simulink model "PhyMtrCtrl"  (R2023b)
settings: Solver=VariableStepAuto  StartTime=0.0  StopTime=10.0  RelTol=1e-3
values from neighbouring files (symbols this model uses):
  B = 0.001889    [MtrCtrl_v01.sldd]    (also in PICal.m; PMSM.m = Simulink.Parameter)
  C_LUT_AngleTable_sng_Null = saveVarsMat.C_LUT_AngleTable_sng_Null    [AngleTable.m]    (also in PMSM.m)
  C_LUT_SinTable_sng_Null = saveVarsMat.C_LUT_SinTable_sng_Null    [AngleTable.m]    (also in PMSM.m)
  C_MATH_OneOverSqrtThree_s32n31_Null = Simulink.Parameter    [PMSM.m]
  C_MATH_Pi_u32n30_Null = Simulink.Parameter    [PMSM.m]
  C_MATH_SqrtThreeOverThree_s32n31_Null = Simulink.Parameter    [PMSM.m]
  C_PMSM_CurQKi_u32n31_null = Simulink.Parameter    [PMSM.m]
  C_PMSM_CurQKp_u32n31_null = Simulink.Parameter    [PMSM.m]
  C_PMSM_Flux_u32n32_Vs = Simulink.Parameter    [PMSM.m]
  Flux = 0.192    [MtrCtrl_v01.sldd]    (also in PICal.m; PMSM.m)
  IBase_A = 2000.0    [MtrCtrl_v01.sldd]    (also in PICal.m = 300; PMSM.m = Simulink.Parameter)
  J = 0.011    [MtrCtrl_v01.sldd]    (also in PICal.m; PMSM.m)
  K_SVM_DefultDuty_s32n31_Null = Simulink.Parameter    [PMSM.m]
  KCCM_VirPosn_flg = 0.0    [MtrCtrl_v01.sldd]    (also in PMSM.m = Simulink.Parameter)
  KCCM_VoltModeEna_Flg = 0.0    [MtrCtrl_v01.sldd]    (also in PMSM.m = Simulink.Parameter)
  Kis = 114583.3333333333    [MtrCtrl_v01.sldd]    (also in PICal.m = 114583.333333; PMSM.m = 114583.333333)
  Kt = 1.1520000000000001    [MtrCtrl_v01.sldd]    (also in PICal.m = 1.152; PMSM.m = 1.152)
  Ld = 80e-6    (= 8e-05)    [FluxweakingGen.m]    (also in IEHB_MAPGenerationtest.m = 6.8e-05; MtrCtrl_v01.sldd = 0.000635; PICal.m = 0.000635; PMSM.m = Simulink.Parameter)
  LPF_coefg = 0.01    [MtrCtrl_v01.sldd]    (also in PMSM.m = Simulink.Parameter)
  Lq = 80e-6    (= 8e-05)    [FluxweakingGen.m]    (also in IEHB_MAPGenerationtest.m = 6e-05; MtrCtrl_v01.sldd = 0.000685; PICal.m = 0.000635; PMSM.m = Simulink.Parameter)
  Ls = 0.000635    [MtrCtrl_v01.sldd]    (also in PICal.m; PMSM.m)
  OneOverUBase_V = Simulink.Parameter    [PMSM.m]
  Pp = 4.0    [MtrCtrl_v01.sldd]    (also in PICal.m = 4; PMSM.m = Simulink.Parameter)
  Rs = 0.03    [FluxweakingGen.m]    (also in MtrCtrl_v01.sldd = 0.05; PICal.m = 0.05; PMSM.m = Simulink.Parameter)
  SecPerRnd = 0.6    [MtrCtrl_v01.sldd]    (also in PMSM.m = Simulink.Parameter)
  sinTable = 0.0015339801862847655 0.0015339807878856412 0.0030679567629659761 0.0030679615757712823 0.0046019261204485705 0.0046019423636569235 0.0061358846491544753 0.0061359231515425647 0.007669828739531097 0.0076699039394282058 0.00920375478205982 0.009203884727313847 0.010737659167264491 0.010737865515199488 0.012271538285719925 0.012271846303085129 0.013805388528060391 0.013805827090970771 0.015339206284    [MtrCtrl_v01.sldd]    (also in SinLut.m = zeros(2,TableSize))
  SMOGain_V = 323.31615074619043    [MtrCtrl_v01.sldd]    (also in PMSM.m = Simulink.Parameter)
  Ts = 0.0001    [MtrCtrl_v01.sldd]    (also in PICal.m; PMSM.m = Simulink.Parameter)
  UBase_V = 600.0    [MtrCtrl_v01.sldd]    (also in PICal.m = 600; PMSM.m = Simulink.Parameter)
  wmBase_rps = 314.15926535897933    [MtrCtrl_v01.sldd]    (also in PICal.m = 314.159265359; PMSM.m = Simulink.Parameter)
undefined symbols (not defined in the file or in its folder): C_PMSM_Ls_pu, C_PMSM_PolePairs_u8_Null, DiscIntNeverNeededParam
libraries: ee_lib x16, simulink x10, nesl_utility x6, spsVoltageMeasurementLib x6, spsCurrentMeasurementLib x3, spsSeriesRLCBranchLib x3, simulink_extras x2, fl_lib x2, sdl_lib x1, eePmsmFwController x1, slpidlib x1, spspowerguiLib x1
(part 2 of 3)

== system PhyMtrCtrl/CurLpCtrl/InversePark ==
  D : Inport  OutDataTypeStr=fixdt(1,32,31)
  Q : Inport  Port=2  OutDataTypeStr=fixdt(1,32,31)
  SinTheta : Inport  Port=3  OutDataTypeStr=fixdt(1,32,30)
  CosTheta : Inport  Port=4  OutDataTypeStr=fixdt(1,32,30)
  Scope : Scope  NumInputPorts=2
  dcos : Product  OutDataTypeStr=fixdt(1,32,31)  RndMeth=Simplest
  dsin : Product  OutDataTypeStr=fixdt(1,32,31)  RndMeth=Simplest
  qcos : Product  OutDataTypeStr=fixdt(1,32,31)  RndMeth=Simplest
  qsin : Product  OutDataTypeStr=fixdt(1,32,31)  RndMeth=Simplest
  sum_alpha : Sum  Inputs=|+-  OutDataTypeStr=fixdt(1,32,31)  RndMeth=Simplest
  sum_beta : Sum  Inputs=|++  OutDataTypeStr=fixdt(1,32,31)  RndMeth=Simplest
  Alpha : Outport
  Beta : Outport  Port=2
  wires:
  sum_alpha/1 -> Scope/1, Alpha/1
  sum_beta/1 -> Scope/2, Beta/1
  dsin/1 -> sum_beta/2
  qcos/1 -> sum_beta/1
  CosTheta/1 -> dcos/2, qcos/2
  qsin/1 -> sum_alpha/2
  SinTheta/1 -> qsin/2, dsin/2
  Q/1 -> qcos/1, qsin/1
  dcos/1 -> sum_alpha/1
  D/1 -> dsin/1, dcos/1

== system PhyMtrCtrl/CurLpCtrl/ParkTF ==
  I_alpha : Inport  OutDataTypeStr=fixdt(1,32,31)
  I_beta : Inport  Port=2  OutDataTypeStr=fixdt(1,32,31)
  SinTheta : Inport  Port=3  OutDataTypeStr=fixdt(1,32,30)
  CosTheta : Inport  Port=4  OutDataTypeStr=fixdt(1,32,30)
  Add : Sum  OutDataTypeStr=fixdt(1,32,31)
  Add1 : Sum  Inputs=+-  OutDataTypeStr=fixdt(1,32,31)
  Product{,1..3} (4 alike) : Product  OutDataTypeStr=fixdt(1,32,31)
  Scope : Scope  NumInputPorts=2
  CurD : Outport
  CurQ : Outport  Port=2
  wires:
  Product/1 -> Add/1
  Product1/1 -> Add/2
  Add/1 -> Scope/1, CurD/1
  Add1/1 -> Scope/2, CurQ/1
  Product3/1 -> Add1/1
  Product2/1 -> Add1/2
  I_alpha/1 -> Product2/1, Product/1
  SinTheta/1 -> Product2/2, Product1/2
  I_beta/1 -> Product1/1, Product3/1
  CosTheta/1 -> Product/2, Product3/2

== system PhyMtrCtrl/CurLpCtrl/PhaseCut ==
  In1 : Inport  OutDataTypeStr=fixdt(1,32,4)
  In2 : Inport  Port=2  OutDataTypeStr=fixdt(0,32,33)
  In3 : Inport  Port=3  OutDataTypeStr=fixdt(0,32,33)
  In4 : Inport  Port=4  OutDataTypeStr=fixdt(0,32,33)
  Constant5 : Constant  Value=0.5  OutDataTypeStr=fixdt(0,32,32)
  Constant6 : Constant  Value=0.0  OutDataTypeStr=fixdt(1,32,4)
  Constant7 : Constant  Value=0.00  OutDataTypeStr=fixdt(1,32,4)
  Switch2 : Switch  Criteria=u2 > Threshold  OutDataTypeStr=fixdt(0,32,33)  SaturateOnIntegerOverflow=off  InputSameDT=off
  Switch3 : Switch  Criteria=u2 > Threshold  OutDataTypeStr=fixdt(0,32,33)  SaturateOnIntegerOverflow=off  InputSameDT=off
  Switch4 : Switch  Criteria=u2 > Threshold  OutDataTypeStr=fixdt(0,32,33)  SaturateOnIntegerOverflow=off  InputSameDT=off
  Out1 : Outport
  Out2 : Outport  Port=2
  Out3 : Outport  Port=3
  wires:
  Switch4/1 -> Out3/1
  Constant7/1 -> Switch4/1
  In2/1 -> Switch2/3
  In1/1 -> Switch2/2, Switch3/2, Switch4/2
  Constant5/1 -> Switch2/1
  Switch2/1 -> Out1/1
  Constant6/1 -> Switch3/1
  Switch3/1 -> Out2/1
  In4/1 -> Switch4/3
  In3/1 -> Switch3/3

== system PhyMtrCtrl/CurLpCtrl/SVPWM ==
  Alpha : Inport  OutDataTypeStr=fixdt(1,32,31)
  Beta : Inport  Port=2  OutDataTypeStr=fixdt(1,32,31)
  Add : Sum  OutDataTypeStr=fixdt(0,32,32)
  Gain : Gain  Gain=1/12  OutDataTypeStr=fixdt(0,32,32)
  Overmodulation : Subsystem
  Scope : Scope
  Scope1 : Scope  NumInputPorts=3
  Scope2 : Scope  NumInputPorts=3
  Scope3 : Scope  NumInputPorts=4
  Scope4 : Scope  NumInputPorts=2
  Sector : Subsystem
  SelectRegion : Subsystem  TreatAsAtomicUnit=on
      settings: RTWSystemCode=Nonreusable function  RTWFcnNameOpts=Use subsystem name
  Sn : Subsystem
  Sqrt : Sqrt  OutDataTypeStr=fixdt(0,32,32)
  Square : Math  Operator=square  OutDataTypeStr=fixdt(1,32,31)
  Square1 : Math  Operator=square  OutDataTypeStr=fixdt(1,32,31)
  SwitchTimeCalculation : Subsystem  TreatAsAtomicUnit=on
      settings: RTWSystemCode=Nonreusable function  RTWFcnNameOpts=Use subsystem name
  TempValueCalculation : Subsystem  TreatAsAtomicUnit=on
      settings: RTWSystemCode=Nonreusable function  RTWFcnNameOpts=Use subsystem name
  Sa : Outport
  Sb : Outport  Port=2
  Sc : Outport  Port=3
  wires:
  Sector/2(Tx) -> Overmodulation/1(Tx), Scope4/1
  Overmodulation/1(Tx_out) -> Sn/2(Tx), Scope3/3
  Overmodulation/2(Ty_out) -> Sn/3(Ty), Scope3/4
  Sector/3(Ty) -> Overmodulation/2(Ty), Scope4/2
  Sector/1(Sector) -> Gain/1, Sn/1(Sector), Scope2/3
  Sn/1(Sa) -> Scope3/1, Sa/1
  Sn/2(Sb) -> Sb/1
  Sn/3(Sc) -> Sc/1
  Gain/1 -> Scope3/2
  SelectRegion/1(N) -> SwitchTimeCalculation/1(N)
  TempValueCalculation/3(V3) -> SelectRegion/3(V3), SwitchTimeCalculation/4(V3)  "V2"
  Alpha/1 -> TempValueCalculation/1(V_alpha), Square/1, Scope2/1, Sector/1(Alpha)
  SwitchTimeCalculation/1(Ta) -> Scope1/1  "Ta"
  TempValueCalculation/2(V2) -> SwitchTimeCalculation/3(V2), SelectRegion/2(V2)  "V3"
  TempValueCalculation/1(V1) -> SwitchTimeCalculation/2(V1), SelectRegion/1(V1)  "V1"
  Beta/1 -> Square1/1, Scope2/2, Sector/2(Beta), TempValueCalculation/2(V_beta)
  SwitchTimeCalculation/3(Tc) -> Scope1/3  "Tc"
  SwitchTimeCalculation/2(Tb) -> Scope1/2  "Tb"
  Add/1 -> Sqrt/1
  Square/1 -> Add/1
  Square1/1 -> Add/2
  Sqrt/1 -> Scope/1

== system PhyMtrCtrl/CurLpCtrl/Subsystem10 ==
  idqRef : Inport  OutDataTypeStr=fixdt(1,32,31)
  vdq : Inport  Port=2  OutDataTypeStr=fixdt(1,32,31)
  VphMax : Inport  Port=3  OutDataTypeStr=fixdt(0,32,32)
  PMSM Field-Weakening Controller : eePmsmFwController/PMSM Field-Weakening Controller  Commented=on  Mth=0.95  Kfw=50  Kaw=10  Ts=-1
  Subsystem : Subsystem
  idqRefFW : Outport
  wires:
  vdq/1 -> Subsystem/2(vdq)
  idqRef/1 -> Subsystem/1(idqRef)
  VphMax/1 -> Subsystem/3(VphMax)
  Subsystem/1(idqRefFW) -> idqRefFW/1

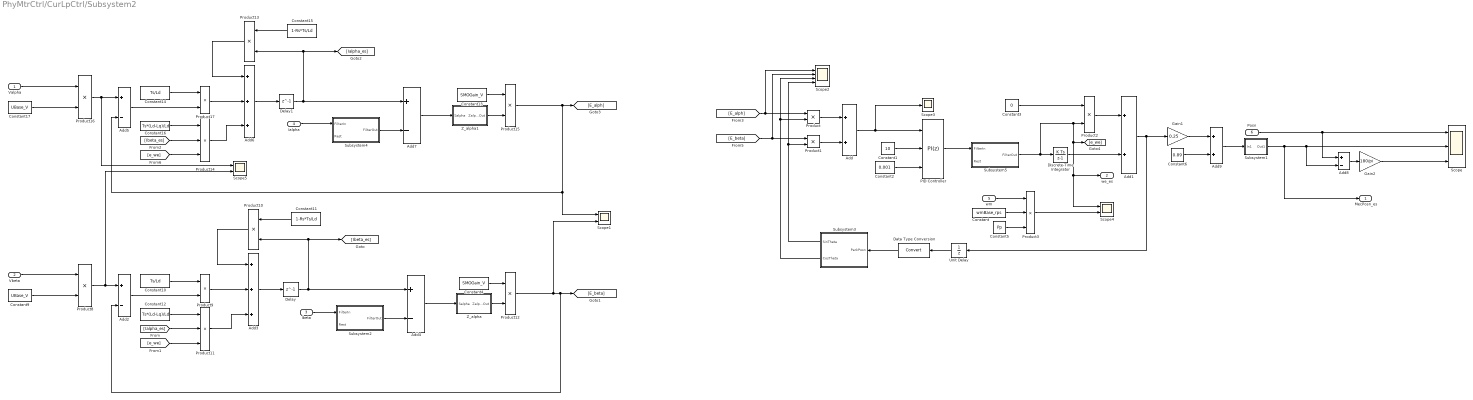
== system PhyMtrCtrl/CurLpCtrl/Subsystem2 ==
  Valpha : Inport  OutDataTypeStr=fixdt(1,32,31)
  Vbeta : Inport  Port=2  OutDataTypeStr=fixdt(1,32,31)
  Ibeta : Inport  Port=3  OutDataTypeStr=fixdt(1,32,31)
  Ialpha : Inport  Port=4  OutDataTypeStr=fixdt(1,32,31)
  wm : Inport  Port=5  OutDataTypeStr=fixdt(1,32,31)
  Posn : Inport  Port=6  OutDataTypeStr=fixdt(1,32,28)
  Add : Sum  OutDataTypeStr=fixdt(1,32,25)
  Add1 : Sum  OutDataTypeStr=fixdt(1,32,24)
  Add2 : Sum  Inputs=+-  OutDataTypeStr=fixdt(1,32,22)
  Add3 : Sum  Inputs=+++  OutDataTypeStr=fixdt(1,32,23)
  Add4 : Sum  Inputs=+-  OutDataTypeStr=int32
  Add5 : Sum  Inputs=+-  OutDataTypeStr=fixdt(1,32,23)
  Add6 : Sum  Inputs=+++  OutDataTypeStr=fixdt(1,32,23)
  Add7 : Sum  Inputs=+-  OutDataTypeStr=fixdt(1,32,0)
  Add8 : Sum  Inputs=+-  OutDataTypeStr=fixdt(1,32,28)
  Add9 : Sum  OutDataTypeStr=fixdt(0,32,0)
  Constant : Constant  Value=wmBase_rps  OutDataTypeStr=fixdt(0,32,23)
  Constant1 : Constant  Value=10  OutDataTypeStr=fixdt(0,32,28)
  Constant10 : Constant  Value=Ts/Ld  OutDataTypeStr=fixdt(0,32,34)
  Constant11 : Constant  Value=1-Rs*Ts/Ld  OutDataTypeStr=fixdt(0,32,32)
  Constant12 : Constant  Value=Ts*(Ld-Lq)/Ld  OutDataTypeStr=fixdt(1,32,47)
  Constant13 : Constant  Value=SMOGain_V  OutDataTypeStr=fixdt(0,32,23)
  Constant14 : Constant  Value=Ts/Ld  OutDataTypeStr=fixdt(0,32,34)
  Constant15 : Constant  Value=1-Rs*Ts/Ld  OutDataTypeStr=fixdt(0,32,32)
  Constant16 : Constant  Value=Ts*(Ld-Lq)/Ld  OutDataTypeStr=fixdt(1,32,47)
  Constant17 : Constant  Value=UBase_V  OutDataTypeStr=fixdt(0,32,22)
  Constant2 : Constant  Value=0.001  OutDataTypeStr=fixdt(0,32,41)
  Constant3 : Constant  Value=0  OutDataTypeStr=fixdt(1,32,4)
  Constant4 : Constant  Value=SMOGain_V  OutDataTypeStr=fixdt(0,32,23)
  Constant5 : Constant  Value=Pp  OutDataTypeStr=fixdt(0,32,29)
  Constant6 : Constant  Value=0.89  OutDataTypeStr=fixdt(0,32,32)
  Constant9 : Constant  Value=UBase_V  OutDataTypeStr=fixdt(0,32,22)
  Data Type Conversion : DataTypeConversion  SaturateOnIntegerOverflow=off  RndMeth=Floor
  Delay : Delay  DelayLength=1
  Delay1 : Delay  DelayLength=1
  Discrete-Time Integrator : DiscreteIntegrator  SampleTime=-1  OutDataTypeStr=fixdt(1,32,24)  ICPrevOutput=DiscIntNeverNeededParam  ICPrevScaledInput=DiscIntNeverNeededParam
  Gain1 : Gain  Gain=0.25  OutDataTypeStr=fixdt(1,32,26)
  Gain2 : Gain  Gain=180/pi  OutDataTypeStr=fixdt(1,32,22)
  PID Controller : slpidlib/PID Controller  Controller=PI  Form=Parallel  TimeDomain=Discrete-time  UseExternalTs=on  SampleTime=-1  IntegratorMethod=Forward Euler  FilterMethod=Forward Euler  ControllerParametersSource=external  P=1  I=1  UseKiTs=on  D=0  N=100  UseFilter=off  TunerSelectOption=Transfer Function Based (PID Tuner App)  InitialConditionSource=internal  InitialConditionForIntegrator=0  InitialConditionForFilter=0  DifferentiatorICPrevScaledInput=0  ExternalReset=none  TrackingMode=off  Kt=1  LimitOutput=off  SatLimitsSource=internal  UpperSaturationLimit=inf  LowerSaturationLimit=-inf  LinearizeAsGain=on  AntiWindupMode=none  Kb=1  LimitIntegrator=off  UpperIntegratorSaturationLimit=inf  LowerIntegratorSaturationLimit=-inf  PGainOutDataTypeStr=fixdt(1,32,22)  PProdOutDataTypeStr=fixdt(1,32,22)  POutMin=[]  POutMax=[]  IGainOutDataTypeStr=fixdt(1,32,35)  IProdOutDataTypeStr=fixdt(1,32,35)  IOutMin=[]  IOutMax=[]  DOutMin=[]  DOutMax=[]  NOutMin=[]  NOutMax=[]  SumOutDataTypeStr=fixdt(1,32,22)  SumOutMin=[]  SumOutMax=[]  SaturationOutMin=[]  SaturationOutMax=[]  PParamMin=[]  PParamMax=[]  IParamMin=[]  IParamMax=[]  DParamMin=[]  DParamMax=[]  NParamMin=[]  NParamMax=[]  KbParamMin=[]  KbParamMax=[]  KtParamMin=[]  KtParamMax=[]  KbOutMin=[]  KbOutMax=[]  KtOutMin=[]  KtOutMax=[]  IntegratorOutDataTypeStr=fixdt(1,32,24)  IntegratorOutMin=[]  IntegratorOutMax=[]  FilterOutMin=[]  FilterOutMax=[]  SumI1OutMin=[]  SumI1OutMax=[]  SumI2OutMin=[]  SumI2OutMax=[]  SumI3OutMin=[]  SumI3OutMax=[]  SumI4OutMin=[]  SumI4OutMax=[]  SumDOutMin=[]  SumDOutMax=[]  DifferentiatorOutMin=[]  DifferentiatorOutMax=[]  FilterDiffOutCoefMin=[]  FilterDiffOutCoefMax=[]  ReciprocalOutMin=[]  ReciprocalOutMax=[]  SumDenOutMin=[]  SumDenOutMax=[]  SumNumOutMin=[]  SumNumOutMax=[]  DivideOutMin=[]  DivideOutMax=[]  UdiffTsProdOutMin=[]  UdiffTsProdOutMax=[]  NTsProdOutMin=[]  NTsProdOutMax=[]  UintegralTsProdOutMin=[]  UintegralTsProdOutMax=[]  UngainTsProdOutMin=[]  UngainTsProdOutMax=[]  ClampingZeroOutDataTypeStr=Inherit: Inherit via back propagation  ClampingZeroOutMin=[]  ClampingZeroOutMax=[]  FilterDenConstantOutDataTypeStr=Inherit: Inherit via back propagation  FilterDenConstantOutMin=[]  FilterDenConstantOutMax=[]  PCopyOutDataTypeStr=Inherit: Inherit via back propagation  PCopyOutMin=[]  PCopyOutMax=[]  NCopyOutDataTypeStr=Inherit: Inherit via back propagation  NCopyOutMin=[]  NCopyOutMax=[]  IntegratorContinuousStateAttributes=''  IntegratorStateMustResolveToSignalObject=off  IntegratorRTWStateStorageClass=Auto  FilterContinuousStateAttributes=''  FilterStateMustResolveToSignalObject=off  FilterRTWStateStorageClass=Auto  ParallelPVariant=ExternalParameters  IdealPVariant=Disabled  IVariant=ExternalParameters  DVariant=Disabled  IntegratorVariant=Discrete  SatVariant=Disabled  AWVariant=Passthrough  PCopyVariant=Disabled  TRVariant=Disabled  FdbkBlocksVariant=Forward  IdealPFdbkVariant=Disabled  SatFdbkVariant=Disabled  DerivativeFilterVariant=Disabled  NVariant=Disabled  NCopyVariant=Disabled_SignalSpec  FilterICVariant=Disabled  IntegratorICVariant=InternalICs  ExternalResetVariant=Disabled  TRSumVariant=Passthrough  SumFdbkVariant=Disabled  SumVariant=Sum_PI  TsampFilterVariant=InternalTs  TsampNgainVariant=Passthrough  TsampIntegralVariant=Passthrough  ExternalSaturationOutDataTypeStr=Inherit: Same as second input
  Product{,1,9,12} (4 alike) : Product  OutDataTypeStr=fixdt(1,32,24)
  Product{10,13,15..16} (4 alike) : Product  OutDataTypeStr=fixdt(1,32,23)
  Product11 : Product  Inputs=3  OutDataTypeStr=fixdt(1,32,31)
  Product14 : Product  Inputs=3  OutDataTypeStr=fixdt(1,32,31)
  Product17 : Product  OutDataTypeStr=fixdt(1,32,26)
  Product2 : Product  OutDataTypeStr=fixdt(1,32,4)
  Product3 : Product  Inputs=3  OutDataTypeStr=fixdt(1,32,23)
  Product8 : Product  OutDataTypeStr=fixdt(1,32,22)
  Scope : Scope  NumInputPorts=3
  Scope1 : Scope  NumInputPorts=2
  Scope2 : Scope  NumInputPorts=4
  Scope3 : Scope
  Scope4 : Scope  NumInputPorts=2
  Scope5 : Scope  NumInputPorts=2
  Subsystem1 : Subsystem
  Subsystem2 : Subsystem
  Subsystem3 : Subsystem
  Subsystem4 : Subsystem
  Subsystem5 : Subsystem
  Unit Delay : UnitDelay  SampleTime=-1  HasFrameUpgradeWarning=on
  Z_alpha : Subsystem
  Z_alpha1 : Subsystem
  MecPosn_es : Outport
  we_es : Outport  Port=2
  wires:
  Valpha/1 -> Product16/1
  Constant9/1 -> Product8/2
  Vbeta/1 -> Product8/1
  Add2/1 -> Product9/2
  Constant10/1 -> Product9/1
  Product9/1 -> Add3/2
  Product10/1 -> Add3/1
  Constant11/1 -> Product10/1
  Add3/1 -> Delay/1
  Delay/1 -> Product10/2, [Ibeta_es], Add4/1
  Product11/1 -> Add3/3
  Constant12/1 -> Product11/1
  [Ialpha_es] -> Product11/2
  [e_we] -> Product11/3
  Ibeta/1 -> Subsystem2/1(FilterIn)
  Subsystem2/1(FilterOut) -> Add4/2
  Add4/1 -> Z_alpha/1(Salpha)
  Z_alpha/1(ZalphaOut) -> Product12/2
  Constant4/1 -> Product12/1
  Product12/1 -> Scope1/2, [E_beta], Add2/2
  Product15/1 -> Add5/2, Scope1/1, [E_alph]
  Constant13/1 -> Product15/1
  Z_alpha1/1(ZalphaOut) -> Product15/2
  Add7/1 -> Z_alpha1/1(Salpha)
  Subsystem4/1(FilterOut) -> Add7/2
  [e_we] -> Product14/3
  [Ibeta_es] -> Product14/2
  Constant16/1 -> Product14/1
  Product14/1 -> Add6/3
  Delay1/1 -> Add7/1, [Ialpha_es], Product13/2
  Constant15/1 -> Product13/1
  Product13/1 -> Add6/1
  Product17/1 -> Add6/2
  Constant14/1 -> Product17/1
  Add5/1 -> Product17/2
  Ialpha/1 -> Subsystem4/1(FilterIn)
  Constant17/1 -> Product16/2
  [E_beta] -> Product1/1, Scope2/2
  Product/1 -> Add/1
  Product1/1 -> Add/2
  Add/1 -> PID Controller/1, Scope3/1
  Constant1/1 -> PID Controller/2
  Constant2/1 -> PID Controller/3
  PID Controller/1 -> Subsystem5/1(FilterIn)
  Discrete-Time Integrator/1 -> Add1/2
  Subsystem5/1(FilterOut) -> [e_we], Scope4/1, we_es/1, Product2/2, Discrete-Time Integrator/1
  Constant3/1 -> Product2/1
  Product2/1 -> Add1/1
  Subsystem3/1(SinTheta) -> Product1/2, Scope2/4
  Subsystem3/2(CosTheta) -> Scope2/3, Product/2
  [E_alph] -> Product/1, Scope2/1
  Add8/1 -> Gain2/1
  wm/1 -> Product3/1
  Constant/1 -> Product3/2
  Add1/1 -> Unit Delay/1, Gain1/1
  Constant5/1 -> Product3/3
  Product3/1 -> Scope4/2
  Gain1/1 -> Add9/1
  Constant6/1 -> Add9/2
  Gain2/1 -> Scope/3
  Add9/1 -> Subsystem1/1(In1)
  Posn/1 -> Scope/1, Add8/1
  Subsystem1/1(Out1) -> Scope/2, Add8/2, MecPosn_es/1
  Unit Delay/1 -> Data Type Conversion/1
  Data Type Conversion/1 -> Subsystem3/1(ParkPosn)
  Add6/1 -> Delay1/1
  Product16/1 -> Add5/1, Scope5/1
  Product8/1 -> Scope5/2, Add2/1

== system PhyMtrCtrl/CurLpCtrl/Subsystem4 ==
  IsSet : Inport  OutDataTypeStr=fixdt(1,32,31)
  FluxDegSet : Inport  Port=2  OutDataTypeStr=fixdt(1,32,4)
  Add : Sum  OutDataTypeStr=fixdt(1,32,4)
  Mux : Mux  Inputs=2
  Product : Product  OutDataTypeStr=fixdt(1,32,31)
  Product1 : Product  OutDataTypeStr=fixdt(1,32,31)
  SinCos : Subsystem  Tag=DecoupledSystem
  pi/2 : Constant  Value=0  OutDataTypeStr=fixdt(1,32,4)
  Idq : Outport
  wires:
  SinCos/2(Out2) -> Product1/1
  SinCos/1(Out1) -> Product/2
  IsSet/1 -> Product1/2, Product/1
  FluxDegSet/1 -> Add/1
  Product/1 -> Mux/1
  Product1/1 -> Mux/2
  Add/1 -> SinCos/1(In1)
  pi/2/1 -> Add/2
  Mux/1 -> Idq/1

== system PhyMtrCtrl/CurLpCtrl/Subsystem5 ==
  ParkPosn : Inport  OutDataTypeStr=fixdt(1,32,28)
  1-D Lookup Table : Lookup_n-D  NumberOfTableDimensions=1  BreakpointsForDimension1=C_LUT_AngleTable_sng_Null  BeginIndexSearchUsingPreviousIndexResult=on  Table=C_LUT_SinTable_sng_Null  ExtrapMethod=Clip  UseLastTableValue=on  ApplyFullPrecisionForLinearInterpolation=on  InternalRulePriority=Speed  OutDataTypeStr=fixdt(0,32,31)  RndMeth=Simplest
  1-D Lookup Table1 : Lookup_n-D  NumberOfTableDimensions=1  BreakpointsForDimension1=C_LUT_AngleTable_sng_Null  BeginIndexSearchUsingPreviousIndexResult=on  Table=C_LUT_SinTable_sng_Null  ExtrapMethod=Clip  UseLastTableValue=on  ApplyFullPrecisionForLinearInterpolation=on  InternalRulePriority=Speed  OutDataTypeStr=fixdt(0,32,31)  RndMeth=Simplest
  Add : Sum  OutDataTypeStr=fixdt(1,32,26)
  Chart : Stateflow chart  TreatAsAtomicUnit=on
  Constant1 : Constant  Value=0  OutDataTypeStr=fixdt(1,32,4)
  Gain : Gain  Gain=4  OutDataTypeStr=fixdt(1,32,26)
  Product : Product  OutDataTypeStr=fixdt(1,32,30)  RndMeth=Simplest
  Product1 : Product  OutDataTypeStr=fixdt(1,32,30)
  Scope : Scope  NumInputPorts=3
  SinTheta : Outport
  CosTheta : Outport  Port=2
  wires:
  ParkPosn/1 -> Gain/1
  Gain/1 -> Add/2
  Constant1/1 -> Add/1
  Product/1 -> Scope/1, SinTheta/1
  Product1/1 -> Scope/2, CosTheta/1
  Add/1 -> Scope/3, Chart/1(Angle)
  Chart/1(SinAngle) -> 1-D Lookup Table/1
  Chart/3(CosAngle) -> 1-D Lookup Table1/1
  1-D Lookup Table/1 -> Product/1
  Chart/2(SinSign) -> Product/2
  1-D Lookup Table1/1 -> Product1/1
  Chart/4(CosSign) -> Product1/2

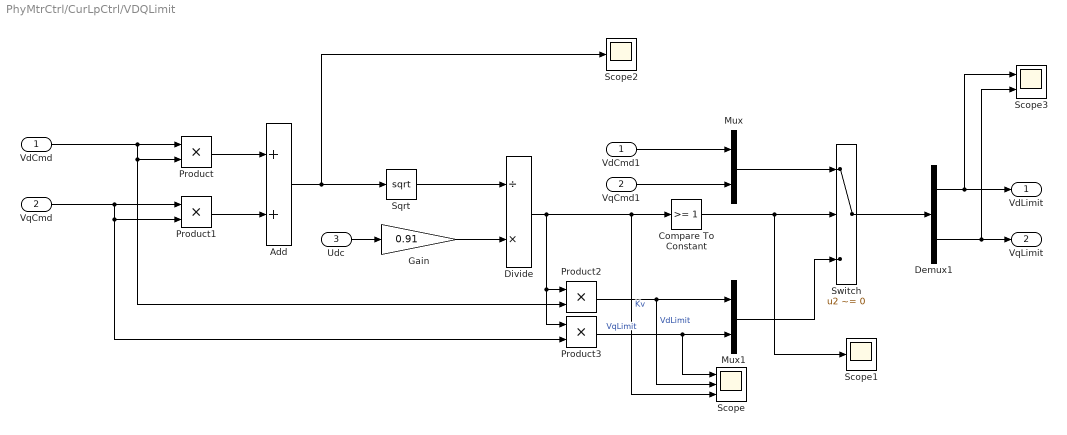
== system PhyMtrCtrl/CurLpCtrl/VDQLimit ==
  VdCmd : Inport  OutDataTypeStr=fixdt(1,32,31)
  VqCmd : Inport  Port=2  OutDataTypeStr=fixdt(1,32,31)
  Udc : Inport  Port=3  OutDataTypeStr=fixdt(0,32,32)
  Add : Sum  OutDataTypeStr=fixdt(0,32,32)
  Compare To Constant : simulink/Logic and Bit Operations/Compare To Constant  relop=>=  const=1  OutDataTypeStr=boolean
  Demux1 : Demux  Outputs=2
  Divide : Product  Inputs=/*  OutDataTypeStr=fixdt(0,32,21)
  Gain : Gain  Gain=0.91  OutDataTypeStr=fixdt(0,32,32)
  Mux : Mux  Inputs=2
  Mux1 : Mux  Inputs=2
  Product : Product  OutDataTypeStr=fixdt(0,32,35)
  Product1 : Product  OutDataTypeStr=fixdt(0,32,33)
  Product2 : Product  OutDataTypeStr=fixdt(1,32,31)
  Product3 : Product  OutDataTypeStr=fixdt(1,32,31)
  Scope : Scope  NumInputPorts=3
  Scope1 : Scope
  Scope2 : Scope
  Scope3 : Scope  NumInputPorts=2
  Sqrt : Sqrt  OutDataTypeStr=fixdt(0,32,32)
  Switch : Switch  Criteria=u2 ~= 0  Threshold=1  OutDataTypeStr=fixdt(1,32,31)  SaturateOnIntegerOverflow=off  InputSameDT=off
  VdCmd1 : InportShadow  OutDataTypeStr=fixdt(1,32,31)
  VqCmd1 : InportShadow  Port=2  OutDataTypeStr=fixdt(1,32,31)
  VdLimit : Outport
  VqLimit : Outport  Port=2
  wires:
  VdCmd/1 -> Product2/2, Product/2, Product/1
  Product/1 -> Add/1
  VqCmd/1 -> Product1/2, Product3/2, Product1/1
  Product1/1 -> Add/2
  Add/1 -> Scope2/1, Sqrt/1
  Sqrt/1 -> Divide/1
  Udc/1 -> Gain/1
  Divide/1 -> Scope/3, Compare To Constant/1, Product2/1, Product3/1  "Kv"
  Compare To Constant/1 -> Scope1/1, Switch/2
  VdCmd1/1 -> Mux/1
  VqCmd1/1 -> Mux/2
  Mux/1 -> Switch/1
  Product2/1 -> Scope/2, Mux1/1  "VdLimit"
  Product3/1 -> Scope/1, Mux1/2  "VqLimit"
  Mux1/1 -> Switch/3
  Switch/1 -> Demux1/1
  Demux1/1 -> Scope3/1, VdLimit/1
  Demux1/2 -> Scope3/2, VqLimit/1
  Gain/1 -> Divide/2

== system PhyMtrCtrl/SpdCtrl/Subsystem1 ==
  Ref : Inport
  Fbk : Inport  Port=2
  Sat : Inport  Port=3
  Add : Sum
  Add1 : Sum  Inputs=+++
  Add2 : Sum  Inputs=+-
  Add3 : Sum
  Gain : Gain  Gain=0.06
  Ki : Constant  Value=1/Kis
  Kp : Constant  Value=1.0
  Kp1 : Constant  Value=0
  Product : Product
  Product1 : Product
  Product2 : Product
  Relational Operator : RelationalOperator  Operator=<=  OutDataTypeStr=boolean  RndMeth=Simplest  InputSameDT=off
  Saturation : Saturate  UpperLimit=220  LowerLimit=-15
  Saturation1 : Saturate  UpperLimit=130  LowerLimit=-15
  Switch : Switch  Criteria=u2 > Threshold  SaturateOnIntegerOverflow=off  InputSameDT=off
  Unit Delay : UnitDelay  SampleTime=-1  HasFrameUpgradeWarning=on
  Unit Delay1 : UnitDelay  SampleTime=-1  HasFrameUpgradeWarning=on
  PIOut : Outport
  wires:
  Kp/1 -> Product/2
  Add1/1 -> PIOut/1
  Product/1 -> Saturation/1
  Add2/1 -> Unit Delay1/1, Add3/1, Product1/2, Product/1
  Add/1 -> Switch/1, Relational Operator/1
  Ki/1 -> Product1/1
  Relational Operator/1 -> Switch/2
  Gain/1 -> Relational Operator/2, Switch/3
  Sat/1 -> Gain/1
  Switch/1 -> Add1/2, Unit Delay/1
  Ref/1 -> Add2/1
  Fbk/1 -> Add2/2
  Saturation/1 -> Add1/1
  Product1/1 -> Add/1
  Unit Delay/1 -> Add/2
  Unit Delay1/1 -> Add3/2
  Add3/1 -> Product2/1
  Kp1/1 -> Product2/2
  Product2/1 -> Saturation1/1
  Saturation1/1 -> Add1/3

== system PhyMtrCtrl/Subsystem/ClarkeTF ==
  Va : Inport
  Vb : Inport  Port=2
  Add : Sum  Inputs=+++
  Gain : Gain  Gain=1/sqrt(3)
  V_alpha : Outport
  V_beta : Outport  Port=2
  wires:
  Add/1 -> Gain/1
  Vb/1 -> Add/3, Add/2
  Va/1 -> V_alpha/1, Add/1
  Gain/1 -> V_beta/1

== system PhyMtrCtrl/Subsystem/InversePark ==
  D : Inport
  Q : Inport  Port=2
  SinTheta : Inport  Port=3
  CosTheta : Inport  Port=4
  Scope : Scope  NumInputPorts=2
  dcos : Product  RndMeth=Simplest  OutDataTypeStr=Inherit: Same as first input
  dsin : Product  RndMeth=Simplest  OutDataTypeStr=Inherit: Same as first input
  qcos : Product  RndMeth=Simplest  OutDataTypeStr=Inherit: Same as first input
  qsin : Product  RndMeth=Simplest  OutDataTypeStr=Inherit: Same as first input
  sum_alpha : Sum  Inputs=|+-  RndMeth=Simplest  OutDataTypeStr=Inherit: Same as first input
  sum_beta : Sum  Inputs=|++  RndMeth=Simplest  OutDataTypeStr=Inherit: Same as first input
  Alpha : Outport
  Beta : Outport  Port=2
  wires:
  sum_alpha/1 -> Scope/1, Alpha/1
  sum_beta/1 -> Scope/2, Beta/1
  dsin/1 -> sum_beta/2
  qcos/1 -> sum_beta/1
  CosTheta/1 -> dcos/2, qcos/2
  qsin/1 -> sum_alpha/2
  SinTheta/1 -> qsin/2, dsin/2
  Q/1 -> qcos/1, qsin/1
  dcos/1 -> sum_alpha/1
  D/1 -> dsin/1, dcos/1

== system PhyMtrCtrl/Subsystem/ParkTF ==
  Valpha : Inport
  Vbeta : Inport  Port=2
  SinTheta : Inport  Port=3
  CosTheta : Inport  Port=4
  Add : Sum
  Add1 : Sum  Inputs=+-
  Product{,1..3} (4 alike) : Product
  Vd : Outport
  Vq : Outport  Port=2
  wires:
  Product/1 -> Add/1
  Product1/1 -> Add/2
  Add/1 -> Vd/1
  Add1/1 -> Vq/1
  Product3/1 -> Add1/1
  Product2/1 -> Add1/2
  Valpha/1 -> Product2/1, Product/1
  SinTheta/1 -> Product2/2, Product1/2
  Vbeta/1 -> Product1/1, Product3/1
  CosTheta/1 -> Product/2, Product3/2

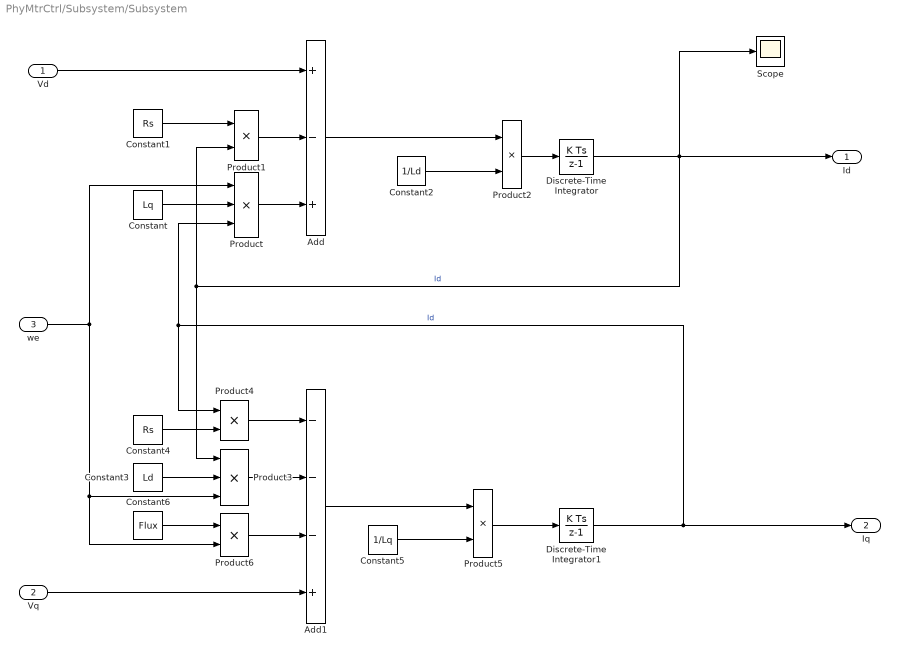
== system PhyMtrCtrl/Subsystem/Subsystem ==
  Vd : Inport
  Vq : Inport  Port=2
  we : Inport  Port=3
  Add : Sum  Inputs=+-+
  Add1 : Sum  Inputs=---+
  Constant : Constant  Value=Lq
  Constant1 : Constant  Value=Rs
  Constant2 : Constant  Value=1/Ld
  Constant3 : Constant  Value=Ld
  Constant4 : Constant  Value=Rs
  Constant5 : Constant  Value=1/Lq
  Constant6 : Constant  Value=Flux
  Discrete-Time Integrator : DiscreteIntegrator  SampleTime=-1  ICPrevOutput=DiscIntNeverNeededParam  ICPrevScaledInput=DiscIntNeverNeededParam
  Discrete-Time Integrator1 : DiscreteIntegrator  SampleTime=-1  ICPrevOutput=DiscIntNeverNeededParam  ICPrevScaledInput=DiscIntNeverNeededParam
  Product : Product  Inputs=3
  Product{1..2,4..6} (5 alike) : Product
  Product3 : Product  Inputs=3
  Scope : Scope
  Id : Outport
  Iq : Outport  Port=2
  wires:
  Discrete-Time Integrator/1 -> Scope/1, Product1/2, Product3/1, Id/1  "Id"
  Vd/1 -> Add/1
  we/1 -> Product6/2, Product3/3, Product/1
  Product5/1 -> Discrete-Time Integrator1/1
  Constant/1 -> Product/2
  Product/1 -> Add/3
  Constant1/1 -> Product1/1
  Product1/1 -> Add/2
  Add/1 -> Product2/1
  Product2/1 -> Discrete-Time Integrator/1
  Constant2/1 -> Product2/2
  Vq/1 -> Add1/4
  Product3/1 -> Add1/2
  Constant3/1 -> Product3/2
  Product4/1 -> Add1/1
  Constant4/1 -> Product4/2
  Constant5/1 -> Product5/2
  Add1/1 -> Product5/1
  Product6/1 -> Add1/3
  Constant6/1 -> Product6/1
  Discrete-Time Integrator1/1 -> Product4/1, Product/3, Iq/1  "Id"

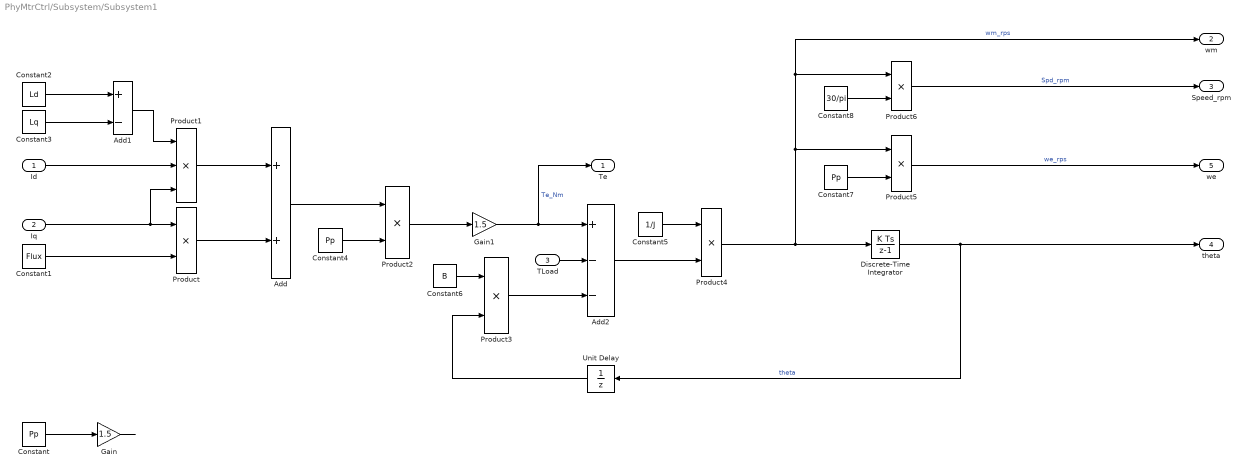
== system PhyMtrCtrl/Subsystem/Subsystem1 ==
  Id : Inport
  Iq : Inport  Port=2
  TLoad : Inport  Port=3
  Add : Sum
  Add1 : Sum  Inputs=+-
  Add2 : Sum  Inputs=+--
  Constant : Constant  Value=Pp
  Constant1 : Constant  Value=Flux
  Constant2 : Constant  Value=Ld
  Constant3 : Constant  Value=Lq
  Constant4 : Constant  Value=Pp
  Constant5 : Constant  Value=1/J
  Constant6 : Constant  Value=B
  Constant7 : Constant  Value=Pp
  Constant8 : Constant  Value=30/pi
  Discrete-Time Integrator : DiscreteIntegrator  SampleTime=-1  ICPrevOutput=DiscIntNeverNeededParam  ICPrevScaledInput=DiscIntNeverNeededParam
  Gain : Gain  Gain=1.5
  Gain1 : Gain  Gain=1.5
  Product{,2..6} (6 alike) : Product
  Product1 : Product  Inputs=3
  Unit Delay : UnitDelay  SampleTime=-1  HasFrameUpgradeWarning=on
  Te : Outport
  wm : Outport  Port=2
  Speed_rpm : Outport  Port=3
  theta : Outport  Port=4
  we : Outport  Port=5
  wires:
  Iq/1 -> Product1/3, Product/1
  Constant/1 -> Gain/1
  Id/1 -> Product1/2
  Constant1/1 -> Product/2
  Gain/1 -> ?
  Product/1 -> Add/2
  Add1/1 -> Product1/1
  Constant2/1 -> Add1/1
  Constant3/1 -> Add1/2
  Product1/1 -> Add/1
  Add/1 -> Product2/1
  Constant4/1 -> Product2/2
  Product2/1 -> Gain1/1
  Gain1/1 -> Add2/1, Te/1  "Te_Nm"
  TLoad/1 -> Add2/2
  Constant7/1 -> Product5/2
  Product5/1 -> we/1  "we_rps"
  Product6/1 -> Speed_rpm/1  "Spd_rpm"
  Constant8/1 -> Product6/2
  Discrete-Time Integrator/1 -> theta/1, Unit Delay/1  "theta"
  Add2/1 -> Product4/2
  Constant5/1 -> Product4/1
  Product4/1 -> Discrete-Time Integrator/1, Product5/1, Product6/1, wm/1  "wm_rps"
  Unit Delay/1 -> Product3/2
  Product3/1 -> Add2/3
  Constant6/1 -> Product3/1

== system PhyMtrCtrl/Subsystem/Subsystem2 ==
  Theta_In : Inport
  Theta_Mtr : Inport  Port=2
  Add : Sum  Inputs=+-
  Constant : Constant  Value=2*pi
  Constant1 : Constant  Value=Pp
  Constant2 : Constant  Value=PosnSelector
  Divide : Product  Inputs=*/  OutDataTypeStr=uint16
  Product : Product
  Product1 : Product
  Scope1 : Scope  NumInputPorts=2
  SinCos : Trigonometry  Operator=sincos
  Switch : Switch  Criteria=u2 > Threshold  SaturateOnIntegerOverflow=off  InputSameDT=off
  SinTheta : Outport
  CoTheta : Outport  Port=2
  wires:
  Theta_In/1 -> Scope1/1, Switch/1
  Constant/1 -> Product1/2, Divide/2
  Divide/1 -> Product1/1
  Add/1 -> SinCos/1
  Product1/1 -> Add/2
  SinCos/1 -> SinTheta/1
  SinCos/2 -> CoTheta/1
  Theta_Mtr/1 -> Scope1/2, Switch/3
  Constant1/1 -> Product/1
  Product/1 -> Add/1, Divide/1
  Switch/1 -> Product/2
  Constant2/1 -> Switch/2

== system PhyMtrCtrl/Subsystem/Subsystem3 ==
  Alpha : Inport
  Beta : Inport  Port=2
  Add : Sum  Inputs=-+
  Add1 : Sum  Inputs=--
  one_by_two : Gain  Gain=1/2  RndMeth=Simplest  OutDataTypeStr=Inherit: Same as input
  sqrt3_by_two : Gain  Gain=sqrt(3)/2  RndMeth=Simplest  OutDataTypeStr=Inherit: Same as input
  CurA : Outport  VectorParamsAs1DForOutWhenUnconnected=off
  CurB : Outport  Port=2  VectorParamsAs1DForOutWhenUnconnected=off
  CurC : Outport  Port=3  VectorParamsAs1DForOutWhenUnconnected=off
  wires:
  sqrt3_by_two/1 -> Add/2, Add1/2
  Add1/1 -> CurC/1
  one_by_two/1 -> Add/1, Add1/1
  Alpha/1 -> CurA/1, one_by_two/1
  Beta/1 -> sqrt3_by_two/1
  Add/1 -> CurB/1

== system PhyMtrCtrl/TqCtrl/Subsystem1 ==
  Ref : Inport
  Fbk : Inport  Port=2
  Sat : Inport  Port=3
  Add : Sum
  Add1 : Sum
  Add2 : Sum  Inputs=+-
  Gain : Gain  Gain=20
  Ki : Constant  Value=0.01
  Kp : Constant  Value=1/Kt
  Product : Product
  Product1 : Product
  Relational Operator : RelationalOperator  Operator=<=  OutDataTypeStr=boolean  RndMeth=Simplest  InputSameDT=off
  Saturation : Saturate  UpperLimit=120  LowerLimit=-130
  Switch : Switch  Criteria=u2 > Threshold  SaturateOnIntegerOverflow=off  InputSameDT=off
  Unit Delay : UnitDelay  SampleTime=-1  HasFrameUpgradeWarning=on
  PIOut : Outport
  wires:
  Kp/1 -> Product/2
  Add1/1 -> PIOut/1
  Product/1 -> Saturation/1
  Add2/1 -> Product1/2, Product/1
  Add/1 -> Switch/1, Relational Operator/1
  Ki/1 -> Product1/1
  Relational Operator/1 -> Switch/2
  Gain/1 -> Relational Operator/2, Switch/3
  Sat/1 -> Gain/1
  Switch/1 -> Add1/2, Unit Delay/1
  Ref/1 -> Add2/1
  Fbk/1 -> Add2/2
  Saturation/1 -> Add1/1
  Product1/1 -> Add/1
  Unit Delay/1 -> Add/2

== system PhyMtrCtrl/CurLpCtrl/CurPILp/Subsystem ==
  IqFb : Inport  OutDataTypeStr=fixdt(1,32,31)
  IdFb : Inport  Port=2  OutDataTypeStr=fixdt(1,32,31)
  wm : Inport  Port=3  OutDataTypeStr=fixdt(1,32,31)
  Enable : EnablePort
  Add : Sum  OutDataTypeStr=fixdt(1,32,31)
  Flux : Constant  Value=C_PMSM_Flux_u32n32_Vs  OutDataTypeStr=fixdt(0,32,32)
  Gain : Gain  Gain=C_PMSM_PolePairs_u8_Null  OutDataTypeStr=fixdt(1,32,31)
  Ld : Gain  Gain=C_PMSM_Ls_pu/4  OutDataTypeStr=fixdt(1,32,31)
  Lq : Gain  Gain=C_PMSM_Ls_pu/2  OutDataTypeStr=fixdt(1,32,31)
  Product : Product  OutDataTypeStr=fixdt(1,32,31)
  Product1 : Product  OutDataTypeStr=fixdt(1,32,31)
  Vdff : Outport
  Vqff : Outport  Port=2
  wires:
  IdFb/1 -> Ld/1
  wm/1 -> Gain/1
  Ld/1 -> Add/1
  Flux/1 -> Add/2
  Add/1 -> Product/1
  Product/1 -> Vqff/1
  IqFb/1 -> Lq/1
  Lq/1 -> Product1/1
  Gain/1 -> Product1/2, Product/2
  Product1/1 -> Vdff/1

== system PhyMtrCtrl/CurLpCtrl/CurPILp/Subsystem1 ==
  Ref : Inport  OutDataTypeStr=fixdt(1,32,31)
  Fbk : Inport  Port=2  OutDataTypeStr=fixdt(1,32,31)
  Sat : Inport  Port=3  OutDataTypeStr=fixdt(0,32,32)
  Add : Sum  OutDataTypeStr=fixdt(1,32,31)
  Add1 : Sum  OutDataTypeStr=fixdt(1,32,31)
  Add2 : Sum  Inputs=+-  OutDataTypeStr=fixdt(1,32,31)
  Gain : Gain  Gain=2/3  OutDataTypeStr=fixdt(0,32,32)
  Ki : Constant  Value=C_PMSM_CurQKi_u32n31_null  OutDataTypeStr=fixdt(0,32,21)
  Kp : Constant  Value=C_PMSM_CurQKp_u32n31_null
  Product : Product  OutDataTypeStr=fixdt(1,32,31)
  Product1 : Product  OutDataTypeStr=fixdt(1,32,31)
  Relational Operator : RelationalOperator  Operator=<=  OutDataTypeStr=boolean  RndMeth=Simplest  InputSameDT=off
  Relational Operator1 : RelationalOperator  Operator=<=  OutDataTypeStr=boolean  RndMeth=Simplest  InputSameDT=off
  Scope : Scope  NumInputPorts=2
  Switch : Switch  Criteria=u2 > Threshold  OutDataTypeStr=fixdt(1,32,31)  SaturateOnIntegerOverflow=off  InputSameDT=off
  Switch1 : Switch  Criteria=u2 > Threshold  OutDataTypeStr=fixdt(1,32,31)  SaturateOnIntegerOverflow=off  InputSameDT=off
  Unit Delay : UnitDelay  SampleTime=-1  HasFrameUpgradeWarning=on
  PIOut : Outport
  wires:
  Ki/1 -> Product/2
  Add1/1 -> PIOut/1
  Add2/1 -> Product/1, Product1/2
  Kp/1 -> Product1/1
  Ref/1 -> Add2/1
  Fbk/1 -> Add2/2
  Product1/1 -> Add/1
  Unit Delay/1 -> Add/2
  Product/1 -> Switch1/1, Relational Operator1/1
  Relational Operator1/1 -> Switch1/2
  Relational Operator/1 -> Switch/2
  Gain/1 -> Switch/3, Switch1/3, Relational Operator1/2, Relational Operator/2
  Sat/1 -> Gain/1
  Switch/1 -> Scope/2, Unit Delay/1, Add1/2
  Switch1/1 -> Scope/1, Add1/1
  Add/1 -> Relational Operator/1, Switch/1

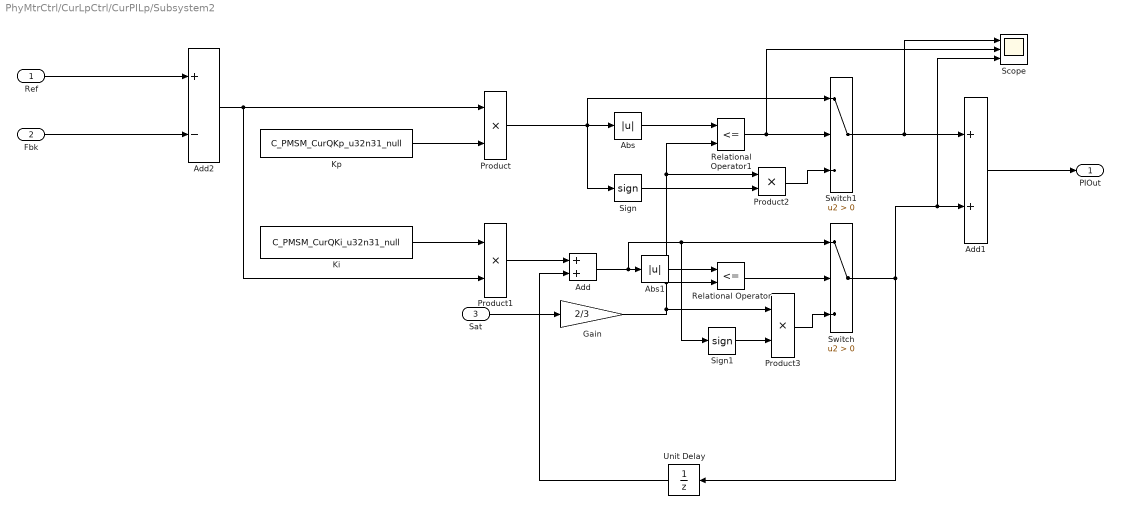
== system PhyMtrCtrl/CurLpCtrl/CurPILp/Subsystem2 ==
  Ref : Inport  OutDataTypeStr=fixdt(1,32,31)
  Fbk : Inport  Port=2  OutDataTypeStr=fixdt(1,32,31)
  Sat : Inport  Port=3  OutDataTypeStr=fixdt(0,32,32)
  Abs : Abs  SaturateOnIntegerOverflow=off
  Abs1 : Abs  SaturateOnIntegerOverflow=off
  Add : Sum  OutDataTypeStr=fixdt(1,32,31)
  Add1 : Sum  OutDataTypeStr=fixdt(1,32,31)
  Add2 : Sum  Inputs=+-  OutDataTypeStr=fixdt(1,32,31)
  Gain : Gain  Gain=2/3  OutDataTypeStr=fixdt(0,32,32)
  Ki : Constant  Value=C_PMSM_CurQKi_u32n31_null  OutDataTypeStr=fixdt(0,32,21)
  Kp : Constant  Value=C_PMSM_CurQKp_u32n31_null
  Product : Product  OutDataTypeStr=fixdt(1,32,31)
  Product1 : Product  OutDataTypeStr=fixdt(1,32,31)
  Product2 : Product
  Product3 : Product
  Relational Operator : RelationalOperator  Operator=<=  OutDataTypeStr=boolean  RndMeth=Simplest  InputSameDT=off
  Relational Operator1 : RelationalOperator  Operator=<=  OutDataTypeStr=boolean  RndMeth=Simplest  InputSameDT=off
  Scope : Scope  NumInputPorts=3
  Sign : Signum
  Sign1 : Signum
  Switch : Switch  Criteria=u2 > Threshold  OutDataTypeStr=fixdt(1,32,31)  SaturateOnIntegerOverflow=off  InputSameDT=off
  Switch1 : Switch  Criteria=u2 > Threshold  OutDataTypeStr=fixdt(1,32,31)  SaturateOnIntegerOverflow=off  InputSameDT=off
  Unit Delay : UnitDelay  SampleTime=-1  HasFrameUpgradeWarning=on
  PIOut : Outport
  wires:
  Add/1 -> Sign1/1, Switch/1, Abs1/1
  Switch1/1 -> Scope/1, Add1/1
  Switch/1 -> Scope/3, Add1/2, Unit Delay/1
  Sat/1 -> Gain/1
  Gain/1 -> Product3/1, Relational Operator/2, Relational Operator1/2, Product2/1
  Relational Operator/1 -> Switch/2
  Relational Operator1/1 -> Scope/2, Switch1/2
  Unit Delay/1 -> Add/2
  Product1/1 -> Add/1
  Fbk/1 -> Add2/2
  Ref/1 -> Add2/1
  Ki/1 -> Product1/1
  Add1/1 -> PIOut/1
  Kp/1 -> Product/2
  Add2/1 -> Product/1, Product1/2
  Product/1 -> Switch1/1, Sign/1, Abs/1
  Abs1/1 -> Relational Operator/1
  Abs/1 -> Relational Operator1/1
  Sign/1 -> Product2/2
  Product2/1 -> Switch1/3
  Sign1/1 -> Product3/2
  Product3/1 -> Switch/3

== system PhyMtrCtrl/CurLpCtrl/CurPILp/Subsystem3 ==
  Vqcmd : Inport  OutDataTypeStr=fixdt(0,32,25)
  Constant6 : Constant  Value=OneOverUBase_V  OutDataTypeStr=fixdt(0,32,32)
  Product : Product  OutDataTypeStr=fixdt(1,32,31)
  Out1 : Outport
  wires:
  Vqcmd/1 -> Product/1
  Constant6/1 -> Product/2
  Product/1 -> Out1/1

== system PhyMtrCtrl/CurLpCtrl/SVPWM/Overmodulation ==
  Tx : Inport  OutDataTypeStr=fixdt(0,32,30)
  Ty : Inport  Port=2  OutDataTypeStr=fixdt(0,32,30)
  Add : Sum  OutDataTypeStr=fixdt(0,32,32)
  Chart : Stateflow chart  TreatAsAtomicUnit=on
  Constant : Constant  OutDataTypeStr=fixdt(0,32,31)
  Constant1 : Constant  Value=0.95  OutDataTypeStr=fixdt(0,32,32)
  Constant2 : Constant  Value=01  OutDataTypeStr=fixdt(0,32,31)
  Data Type Conversion : DataTypeConversion  SaturateOnIntegerOverflow=off  RndMeth=Floor
  Data Type Conversion1 : DataTypeConversion  SaturateOnIntegerOverflow=off  RndMeth=Floor
  Data Type Conversion2 : DataTypeConversion  SaturateOnIntegerOverflow=off  RndMeth=Floor
  Product2 : Product  OutDataTypeStr=fixdt(0,32,32)
  Scope : Scope  NumInputPorts=5
  Subsystem2 : Subsystem
  Switch : Switch  Criteria=u2 > Threshold  OutDataTypeStr=fixdt(0,32,33)  SaturateOnIntegerOverflow=off  InputSameDT=off
  Switch1 : Switch  Criteria=u2 > Threshold  OutDataTypeStr=fixdt(0,32,33)  SaturateOnIntegerOverflow=off  InputSameDT=off
  Tx_out : Outport
  Ty_out : Outport  Port=2
  wires:
  Constant1/1 -> Product2/2
  Constant/1 -> Product2/1
  Tx/1 -> Scope/2, Add/1, Chart/2(Ty), Subsystem2/2(Tx)
  Ty/1 -> Scope/3, Add/2, Chart/3(Tx), Subsystem2/3(Ty)
  Product2/1 -> Data Type Conversion2/1, Subsystem2/1(Ts)
  Subsystem2/1(Tx_o) -> Switch/1
  Chart/1(Tx_o) -> Data Type Conversion1/1
  Switch/1 -> Scope/4, Tx_out/1
  Switch1/1 -> Scope/5, Ty_out/1
  Subsystem2/2(Ty_o) -> Switch1/1
  Chart/2(Ty_o) -> Data Type Conversion/1
  Constant2/1 -> Switch1/2, Switch/2
  Add/1 -> Scope/1
  Data Type Conversion/1 -> Switch1/3
  Data Type Conversion1/1 -> Switch/3
  Data Type Conversion2/1 -> Chart/1(Ts)

== system PhyMtrCtrl/CurLpCtrl/SVPWM/Sector ==
  Alpha : Inport  OutDataTypeStr=fixdt(1,32,31)
  Beta : Inport  Port=2  OutDataTypeStr=fixdt(1,32,31)
  Add : Sum  Inputs=-+  OutDataTypeStr=fixdt(1,32,31)
  Add1 : Sum  Inputs=--  OutDataTypeStr=fixdt(1,32,31)
  Add2 : Sum  Inputs=3  OutDataTypeStr=fixdt(0,32,29)
  Chart : Stateflow chart  TreatAsAtomicUnit=on
  Compare To Constant : simulink/Logic and Bit Operations/Compare To Constant  relop=>  const=0  OutDataTypeStr=uint8
  Compare To Constant1 : simulink/Logic and Bit Operations/Compare To Constant  relop=>  const=0  OutDataTypeStr=uint8
  Compare To Constant2 : simulink/Logic and Bit Operations/Compare To Constant  relop=>  const=0  OutDataTypeStr=uint8
  Constant : Constant  Commented=on  Value=1/UBase_V
  Data Type Conversion : DataTypeConversion  SaturateOnIntegerOverflow=off  RndMeth=Floor
  Data Type Conversion1 : DataTypeConversion  SaturateOnIntegerOverflow=off  RndMeth=Floor
  Gain : Gain  Gain=2  OutDataTypeStr=fixdt(0,32,30)
  Gain1 : Gain  Gain=4  OutDataTypeStr=fixdt(0,32,29)
  Product : Product  Commented=on
  Product1 : Product  Commented=on
  Scope3 : Scope
  one_by_two : Gain  Gain=1/2  OutDataTypeStr=fixdt(1,32,31)  RndMeth=Simplest
  sqrt3_by_two : Gain  Gain=sqrt(3)/2  OutDataTypeStr=fixdt(1,32,31)  RndMeth=Simplest
  Sector : Outport
  Tx : Outport  Port=2
  Ty : Outport  Port=3
  wires:
  Add1/1 -> Compare To Constant2/1, Chart/3(Uc)
  Add/1 -> Compare To Constant1/1, Chart/2(Ub)
  one_by_two/1 -> Add1/1, Add/1
  sqrt3_by_two/1 -> Add1/2, Add/2
  Compare To Constant/1 -> Add2/1
  Compare To Constant1/1 -> Gain/1
  Compare To Constant2/1 -> Gain1/1
  Chart/1(Sector) -> Sector/1
  Gain/1 -> Add2/2
  Gain1/1 -> Add2/3
  Add2/1 -> Chart/4(N), Scope3/1  "N"
  Chart/2(Tx) -> Data Type Conversion/1
  Chart/3(Ty) -> Data Type Conversion1/1
  Beta/1 -> Chart/1(Ua), Compare To Constant/1, one_by_two/1
  Alpha/1 -> sqrt3_by_two/1
  Constant/1 -> Product1/2, Product/2
  Data Type Conversion/1 -> Tx/1
  Data Type Conversion1/1 -> Ty/1

== system PhyMtrCtrl/CurLpCtrl/SVPWM/SelectRegion ==
  V1 : Inport  OutDataTypeStr=fixdt(1,32,31)
  V2 : Inport  Port=2  OutDataTypeStr=fixdt(1,32,32)
  V3 : Inport  Port=3  OutDataTypeStr=fixdt(1,32,32)
  A : Switch  Criteria=u2 > Threshold  OutDataTypeStr=fixdt(0,32,30)  RndMeth=Zero  SaturateOnIntegerOverflow=off  InputSameDT=off
  B : Switch  Criteria=u2 > Threshold  OutDataTypeStr=fixdt(0,32,29)  RndMeth=Zero  SaturateOnIntegerOverflow=off  InputSameDT=off
  C : Switch  Criteria=u2 > Threshold  OutDataTypeStr=fixdt(0,32,30)  RndMeth=Zero  SaturateOnIntegerOverflow=off  InputSameDT=off
  Constant1 : Constant  OutDataTypeStr=fixdt(0,32,30)
  Constant2 : Constant  OutDataTypeStr=fixdt(0,32,30)
  Constant3 : Constant  Value=3  OutDataTypeStr=fixdt(0,32,30)
  Constant4 : Constant  Value=7  OutDataTypeStr=fixdt(0,32,29)
  Sum : Sum  Inputs=-+|  OutDataTypeStr=fixdt(0,32,30)
  Sum1 : Sum  Inputs=|-+  OutDataTypeStr=fixdt(0,32,29)  AccumDataTypeStr=fixdt(0,32,29)
  Sum2 : Sum  Inputs=-+|  OutDataTypeStr=fixdt(0,32,30)
  N : Outport
  wires:
  B/1 -> N/1
  V2/1 -> A/2
  Constant3/1 -> A/3, Sum/2
  Constant1/1 -> Sum/1
  Sum/1 -> A/1
  V3/1 -> C/2
  V1/1 -> B/2
  A/1 -> C/3, Sum2/2
  Constant2/1 -> Sum2/1
  Sum2/1 -> C/1
  C/1 -> B/1, Sum1/1
  Sum1/1 -> B/3
  Constant4/1 -> Sum1/2

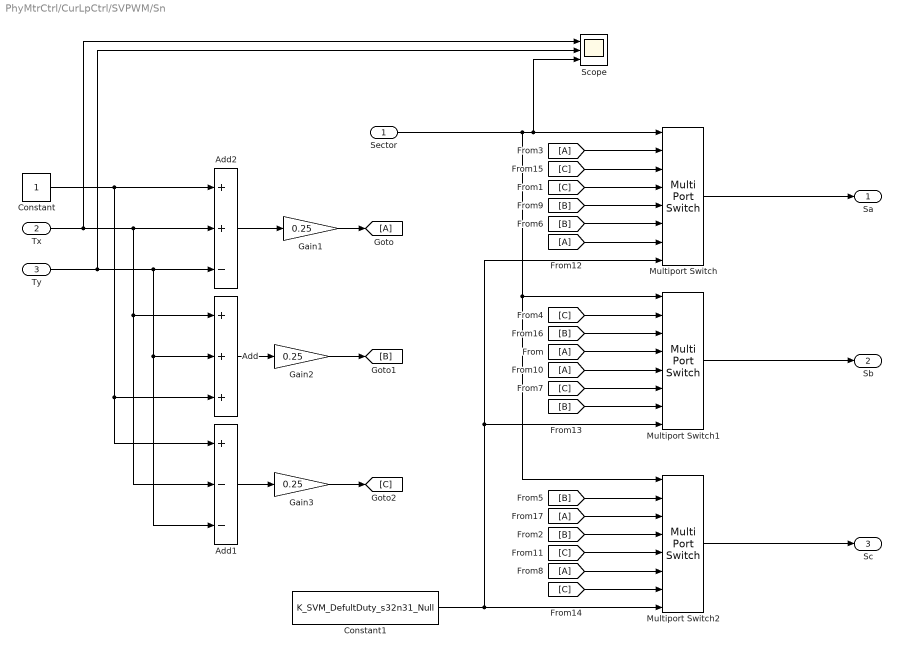
== system PhyMtrCtrl/CurLpCtrl/SVPWM/Sn ==
  Sector : Inport  OutDataTypeStr=uint8
  Tx : Inport  Port=2  OutDataTypeStr=fixdt(0,32,33)
  Ty : Inport  Port=3  OutDataTypeStr=fixdt(0,32,33)
  Add : Sum  Inputs=+++  OutDataTypeStr=fixdt(0,32,31)
  Add1 : Sum  Inputs=+--  OutDataTypeStr=fixdt(0,32,31)
  Add2 : Sum  Inputs=++-  OutDataTypeStr=fixdt(0,32,31)
  Constant : Constant  OutDataTypeStr=fixdt(0,32,31)
  Constant1 : Constant  Value=K_SVM_DefultDuty_s32n31_Null
  From{,3,8,10,12,17} (6 alike) : From
  Gain1 : Gain  Gain=0.25  OutDataTypeStr=fixdt(0,32,33)
  Gain2 : Gain  Gain=0.25  OutDataTypeStr=fixdt(0,32,33)
  Gain3 : Gain  Gain=0.25  OutDataTypeStr=fixdt(0,32,33)
  Goto : Goto
  Multiport Switch : MultiPortSwitch  Inputs=6  DataPortForDefault=Additional data port  OutDataTypeStr=fixdt(0,32,33)  SaturateOnIntegerOverflow=off  InputSameDT=off
  Multiport Switch1 : MultiPortSwitch  Inputs=6  DataPortForDefault=Additional data port  OutDataTypeStr=fixdt(0,32,33)  SaturateOnIntegerOverflow=off  InputSameDT=off
  Multiport Switch2 : MultiPortSwitch  Inputs=6  DataPortForDefault=Additional data port  OutDataTypeStr=fixdt(0,32,33)  SaturateOnIntegerOverflow=off  InputSameDT=off
  Scope : Scope  NumInputPorts=3
  Sa : Outport
  Sb : Outport  Port=2
  Sc : Outport  Port=3
  wires:
  Tx/1 -> Scope/1, Add1/2, Add/1, Add2/2
  Ty/1 -> Scope/2, Add1/3, Add/2, Add2/3
  Add/1 -> Gain2/1
  Constant/1 -> Add1/1, Add/3, Add2/1
  Add2/1 -> Gain1/1
  Add1/1 -> Gain3/1
  Sector/1 -> Multiport Switch/1, Scope/3, Multiport Switch2/1, Multiport Switch1/1
  Multiport Switch/1 -> Sa/1
  Multiport Switch1/1 -> Sb/1
  Multiport Switch2/1 -> Sc/1
  Gain1/1 -> Goto/1
  Gain2/1 -> [B]
  Gain3/1 -> [C]
  [C] -> Multiport Switch/4
  From/1 -> Multiport Switch1/4
  [B] -> Multiport Switch2/4
  From3/1 -> Multiport Switch/2
  [C] -> Multiport Switch1/2
  [B] -> Multiport Switch2/2
  [B] -> Multiport Switch/6
  [C] -> Multiport Switch1/6
  From8/1 -> Multiport Switch2/6
  [B] -> Multiport Switch/5
  From10/1 -> Multiport Switch1/5
  [C] -> Multiport Switch2/5
  From12/1 -> Multiport Switch/7
  [B] -> Multiport Switch1/7
  [C] -> Multiport Switch2/7
  [C] -> Multiport Switch/3
  [B] -> Multiport Switch1/3
  From17/1 -> Multiport Switch2/3
  Constant1/1 -> Multiport Switch/8, Multiport Switch1/8, Multiport Switch2/8

== system PhyMtrCtrl/CurLpCtrl/SVPWM/SwitchTimeCalculation ==
  N : Inport  OutDataTypeStr=fixdt(0,32,29)
  V1 : Inport  Port=2  OutDataTypeStr=fixdt(1,32,31)
  V2 : Inport  Port=3  OutDataTypeStr=fixdt(1,32,32)
  V3 : Inport  Port=4  OutDataTypeStr=fixdt(1,32,32)
  A : MultiPortSwitch  Inputs=6  OutDataTypeStr=fixdt(1,32,32)  SaturateOnIntegerOverflow=off  InputSameDT=off
  B : MultiPortSwitch  Inputs=6  OutDataTypeStr=fixdt(1,32,31)  SaturateOnIntegerOverflow=off  InputSameDT=off
  C : MultiPortSwitch  Inputs=6  OutDataTypeStr=fixdt(1,32,31)  SaturateOnIntegerOverflow=off  InputSameDT=off
  Gain1 : Gain  Gain=-1  ParamDataTypeStr=fixdt(1,32,31)  OutDataTypeStr=fixdt(1,32,32)
  Gain2 : Gain  Gain=-1  ParamDataTypeStr=fixdt(1,32,31)  OutDataTypeStr=fixdt(1,32,31)
  Gain3 : Gain  Gain=-1  ParamDataTypeStr=fixdt(1,32,31)  OutDataTypeStr=fixdt(1,32,32)
  Sum : Sum  Inputs=|++  OutDataTypeStr=fixdt(1,32,32)  AccumDataTypeStr=fixdt(1,32,32)
  Sum1 : Sum  Inputs=-+|  OutDataTypeStr=fixdt(1,32,30)  AccumDataTypeStr=fixdt(1,32,30)
  Sum2 : Sum  Inputs=|++  OutDataTypeStr=fixdt(1,32,30)  AccumDataTypeStr=fixdt(1,32,30)
  Ta : Outport
  Tb : Outport  Port=2
  Tc : Outport  Port=3
  wires:
  N/1 -> A/1, B/1, C/1
  A/1 -> Ta/1
  B/1 -> Tb/1
  C/1 -> Tc/1
  V2/1 -> Gain1/1, A/2, A/5, Sum/1
  V3/1 -> Gain3/1, A/7, A/4, Sum/2, Sum1/1
  Sum/1 -> A/6, A/3
  V1/1 -> Gain2/1, B/3, B/6, Sum1/2
  Sum1/1 -> B/2, B/5
  Gain3/1 -> B/4, B/7
  Gain1/1 -> C/5, C/2, Sum2/1
  Gain2/1 -> C/3, C/6, Sum2/2
  Sum2/1 -> C/7, C/4

== system PhyMtrCtrl/CurLpCtrl/SVPWM/TempValueCalculation ==
  V_alpha : Inport  OutDataTypeStr=fixdt(1,32,31)
  V_beta : Inport  Port=2  OutDataTypeStr=fixdt(1,32,31)
  Add : Sum  Inputs=+-  OutDataTypeStr=fixdt(1,32,32)
  Add1 : Sum  OutDataTypeStr=fixdt(1,32,32)
  Gain : Gain  Gain=0.5  OutDataTypeStr=fixdt(1,32,32)
  Gain1 : Gain  Gain=sqrt(3)/2  OutDataTypeStr=fixdt(1,32,33)
  V1 : Outport  VectorParamsAs1DForOutWhenUnconnected=off
  V2 : Outport  Port=2  VectorParamsAs1DForOutWhenUnconnected=off
  V3 : Outport  Port=3  VectorParamsAs1DForOutWhenUnconnected=off
  wires:
  V_alpha/1 -> Gain1/1
  Gain1/1 -> Add1/2
  Add1/1 -> V2/1, Add/1  "V2"
  V_beta/1 -> Gain/1, Add/2, V1/1  "V1"
  Add/1 -> V3/1  "V3"
  Gain/1 -> Add1/1

== system PhyMtrCtrl/CurLpCtrl/Subsystem10/Subsystem ==
  idqRef : Inport  OutDataTypeStr=fixdt(1,32,31)
  vdq : Inport  Port=2  OutDataTypeStr=fixdt(1,32,31)
  VphMax : Inport  Port=3  OutDataTypeStr=fixdt(0,32,32)
  Cartesian to Polar : Subsystem  Tag=DecoupledSystem
  Constant : Constant  Value=C_MATH_Pi_u32n30_Null  OutDataTypeStr=fixdt(0,32,30)  SampleTime=-1
  Demux : Demux  Outputs=2
  Discrete-Time Integrator : DiscreteIntegrator  IntegratorMethod=Integration: Backward Euler  gainval=5  InitialCondition=1  SampleTime=-1  OutDataTypeStr=fixdt(1,32,28)  ICPrevOutput=DiscIntNeverNeededParam  ICPrevScaledInput=DiscIntNeverNeededParam
  Gain : Gain  Gain=50  OutDataTypeStr=fixdt(1,32,25)
  Gain1 : Gain  Gain=10  OutDataTypeStr=fixdt(1,32,25)
  Gain2 : Gain  Gain=2
  Modulation index threshold : Constant  Value=C_MATH_SqrtThreeOverThree_s32n31_Null  OutDataTypeStr=fixdt(0,32,31)  SampleTime=-1
  Modulation index threshold1 : Constant  Value=3.24  OutDataTypeStr=fixdt(0,32,30)  SampleTime=-1
  Mux : Mux  Inputs=2
  Polar to Cartesian : Subsystem  Tag=DecoupledSystem
  Product : Product  OutDataTypeStr=fixdt(1,32,28)
  Saturation : Saturate  UpperLimit=1  LowerLimit=0  OutDataTypeStr=fixdt(1,32,28)
  Subsystem1 : Subsystem
  Sum : Sum  Inputs=|-+  OutDataTypeStr=fixdt(1,32,30)
  Sum1 : Sum  Inputs=|-+  OutDataTypeStr=fixdt(1,32,28)
  Sum2 : Sum  Inputs=|-+  OutDataTypeStr=fixdt(1,32,28)
  Sum3 : Sum  Inputs=-+  OutDataTypeStr=fixdt(1,32,28)
  Sum4 : Sum  Inputs=|++  OutDataTypeStr=fixdt(1,32,25)
  Unit Delay : UnitDelay  SampleTime=-1  HasFrameUpgradeWarning=on
  idqRefFW : Outport  VectorParamsAs1DForOutWhenUnconnected=off
  wires:
  Product/1 -> Sum2/1
  Sum1/1 -> Product/1
  Gain1/1 -> Sum4/2
  Cartesian to Polar/1(Out1) -> Polar to Cartesian/1(In1)
  Subsystem1/1(M) -> Sum/1
  Sum/1 -> Gain/1
  Discrete-Time Integrator/1 -> Saturation/1, Sum3/1
  Unit Delay/1 -> Gain1/1
  Cartesian to Polar/2(Out2) -> Sum1/1
  Polar to Cartesian/2(Out2) -> Mux/2
  Mux/1 -> idqRefFW/1
  Gain/1 -> Sum4/1
  VphMax/1 -> Subsystem1/2(VphMax)
  Modulation index threshold/1 -> Gain2/1
  Saturation/1 -> Product/2, Sum3/2
  Demux/2 -> Cartesian to Polar/2(In2)
  Demux/1 -> Cartesian to Polar/1(In1)
  idqRef/1 -> Demux/1
  Polar to Cartesian/1(Out1) -> Mux/1
  Constant/1 -> Sum1/2, Sum2/2
  Sum3/1 -> Unit Delay/1
  vdq/1 -> Subsystem1/1(vdq)
  Sum2/1 -> Polar to Cartesian/2(In2)
  Sum4/1 -> Discrete-Time Integrator/1
  Gain2/1 -> Sum/2

== system PhyMtrCtrl/CurLpCtrl/Subsystem2/Subsystem1 ==
  In1 : Inport  OutDataTypeStr=fixdt(0,32,0)
  Constant7 : Constant  Value=2*pi  OutDataTypeStr=fixdt(0,32,0)
  Mod : Math  Operator=mod
  Out1 : Outport
  wires:
  Mod/1 -> Out1/1
  In1/1 -> Mod/1
  Constant7/1 -> Mod/2

== system PhyMtrCtrl/CurLpCtrl/Subsystem2/Subsystem2 ==
  FilterIn : Inport  OutDataTypeStr=fixdt(1,32,31)
  Rest : Inport  Port=2  OutDataTypeStr=fixdt(1,32,0)
  Add : Sum  Inputs=+-  OutDataTypeStr=fixdt(1,32,31)
  Add1 : Sum  OutDataTypeStr=fixdt(1,32,31)
  Constant : Constant  Value=LPF_coefg  OutDataTypeStr=fixdt(0,32,31)
  Delay : Delay  DelayLength=1  ExternalReset=Either
      settings: InputPortMap=u0,r5
  Product : Product  OutDataTypeStr=fixdt(1,32,31)
  FilterOut : Outport
  wires:
  FilterIn/1 -> Add/1
  Add/1 -> Product/2
  Product/1 -> Add1/1
  Add1/1 -> Delay/1, FilterOut/1
  Delay/1 -> Add/2, Add1/2
  Rest/1 -> Delay/2
  Constant/1 -> Product/1
